simulink model "ignitionScheduler"  (R2020b)
settings: Solver=VariableStepAuto  StartTime=0.0  StopTime=30  RelTol=1e-3
undefined symbols (not defined in the file): I, initialize, T, terminate
libraries: simulink x1, SignalEditorBlockLib x1
settings Model: PauseTimes=75  Creator=Guy  LastModifiedBy=sanumula
settings DataIOCC: SaveOutput=off  DSMLogging=off  SaveTime=off
settings OptimizationCC: UseDivisionForNetSlopeComputation=on
settings DebuggingCC: PregeneratedLibrarySubsystemCodeDiagnostic=none  ArithmeticOperatorsInVariantConditions=warning
settings ModelReferenceCC: EnableRefExpFcnMdlSchedulingChecks=off
settings SFSimCC: SimUseLocalCustomCode=off  CustomCodeUndefinedFunction=UseInterfaceOnly
settings RTWCC: RTWUseLocalCustomCode=off
settings SimscapeCC: SimscapeNormalizeSystem=off  SimscapeLogSimulationStatistics=on  SimscapeLogLimitData=off

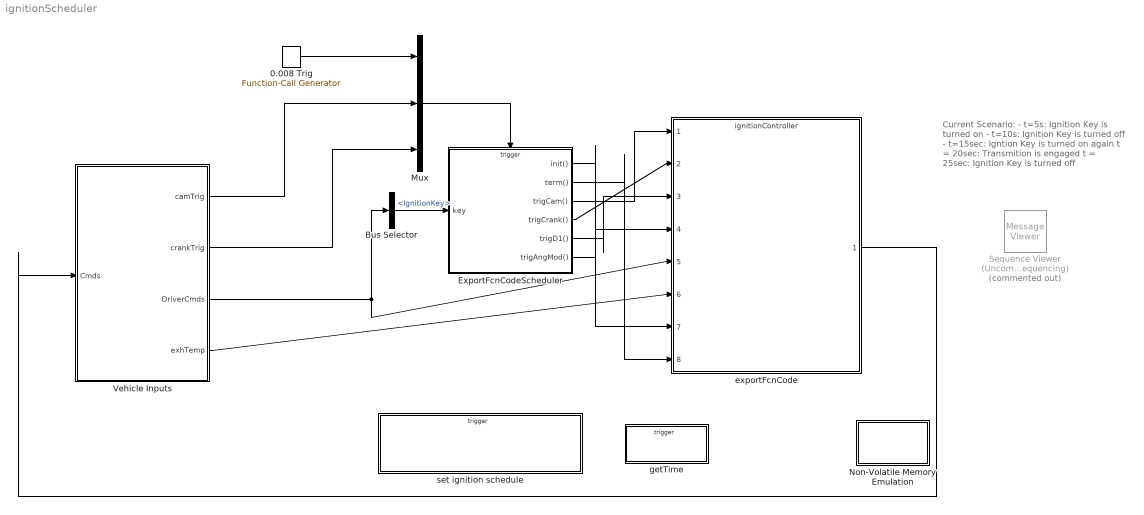
== system ignitionScheduler ==
  note: Current Scenario:
      | - t=5s: Ignition Key is turned on
      | - t=10s: Ignition Key is turned off
      | - t=15sec: Igntion Key is turned on again
      | t = 20sec: Transmition is engaged
      | t = 25sec: Ignition Key is turned off
  0.008 Trig : simulink/Ports & Subsystems/Function-Call Generator  sample_time=.008  numberOfIterations=1  DisallowWideOutput=off
  Bus Selector : BusSelector  OutputSignals=IgnitionKey
  ExportFcnCodeScheduler : Stateflow chart  TreatAsAtomicUnit=on
  Mux : Mux  Inputs=3
  Non-Volatile Memory Emulation : Subsystem
  Sequence Viewer (Uncomment to view events sequencing) : MessageViewer  Commented=on
  Vehicle Inputs : Subsystem
  exportFcnCode : ModelReference  ModelNameDialog=ignitionController.slx  SimulationMode=Normal  ShowModelInitializePort=on  ShowModelTerminatePort=on  ScheduleRates=on  ModelEventPortInfo=I:initialize,T:terminate  ModelReferenceVersion=1.1
  getTime : Subsystem  TreatAsAtomicUnit=on
  set ignition schedule : Subsystem  TreatAsAtomicUnit=on
  wires:
  0.008 Trig/1 -> Mux/1
  Mux/1 -> ExportFcnCodeScheduler/Trigger
  Vehicle Inputs/1(camTrig) -> Mux/2
  Vehicle Inputs/2(crankTrig) -> Mux/3
  Bus Selector/1 -> ExportFcnCodeScheduler/1(key)  "<IgnitionKey>"
  exportFcnCode/1 -> Vehicle Inputs/1(Cmds)
  ExportFcnCodeScheduler/1(init()) -> exportFcnCode/7
  ExportFcnCodeScheduler/2(term()) -> exportFcnCode/8
  ExportFcnCodeScheduler/3(trigCam()) -> exportFcnCode/1
  ExportFcnCodeScheduler/4(trigCrank()) -> exportFcnCode/2
  ExportFcnCodeScheduler/5(trigD1()) -> exportFcnCode/3
  Vehicle Inputs/3(DriverCmds) -> Bus Selector/1, exportFcnCode/5
  Vehicle Inputs/4(exhTemp) -> exportFcnCode/6
  ExportFcnCodeScheduler/6(trigAngMod()) -> exportFcnCode/4

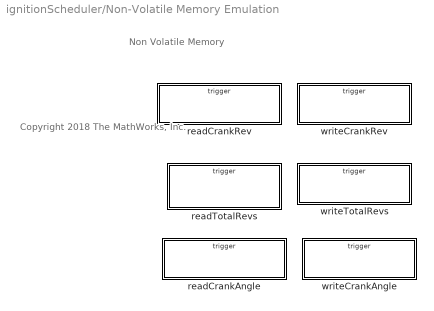
== system ignitionScheduler/Non-Volatile Memory Emulation ==
  note: Copyright 2018 The MathWorks, Inc.
  note: Non Volatile Memory
  readCrankAngle : Subsystem  TreatAsAtomicUnit=on
  readCrankRev : Subsystem  TreatAsAtomicUnit=on
  readTotalRevs : Subsystem  TreatAsAtomicUnit=on
  writeCrankAngle : Subsystem  TreatAsAtomicUnit=on
  writeCrankRev : Subsystem  TreatAsAtomicUnit=on
  writeTotalRevs : Subsystem  TreatAsAtomicUnit=on

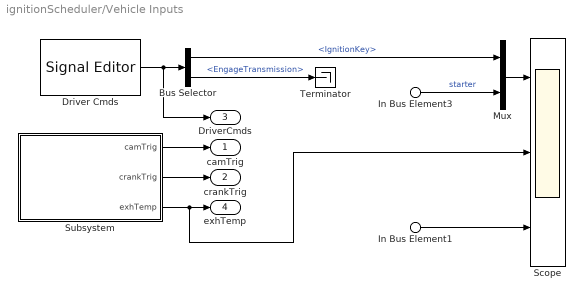
== system ignitionScheduler/Vehicle Inputs ==
  In Bus Element1 : Inport  PortName=Cmds  Element=throttle
  In Bus Element3 : Inport  PortName=Cmds  Element=starter
  Bus Selector : BusSelector  OutputSignals=IgnitionKey,EngageTransmission
  Driver Cmds : SignalEditorBlockLib/Signal Editor  FileName=inputScenarios.mat  ActiveScenario=StartStopTwice  ActiveSignal=CmdBus  IsBus=on  OutputBusObjectStr=Bus: opCmdBus  SampleTime=0  Interpolate=off  ZeroCross=off  OutputAfterFinalValue=Setting to zero  Unit=inherit  PreserveSignalName=on
  Mux : Mux  Inputs=2
  Scope : Scope  NumInputPorts=3
  Subsystem : Subsystem
  Terminator : Terminator
  camTrig : Outport  VectorParamsAs1DForOutWhenUnconnected=off
  crankTrig : Outport  Port=2  VectorParamsAs1DForOutWhenUnconnected=off
  DriverCmds : Outport  Port=3  VectorParamsAs1DForOutWhenUnconnected=off
  exhTemp : Outport  Port=4  VectorParamsAs1DForOutWhenUnconnected=off
  wires:
  Driver Cmds/1 -> DriverCmds/1, Bus Selector/1
  Bus Selector/2 -> Terminator/1  "<EngageTransmission>"
  Mux/1 -> Scope/1
  In Bus Element1/1 -> Scope/3
  In Bus Element3/1 -> Mux/2  "starter"
  Bus Selector/1 -> Mux/1  "<IgnitionKey>"
  Subsystem/1(camTrig) -> camTrig/1
  Subsystem/2(crankTrig) -> crankTrig/1
  Subsystem/3(exhTemp) -> Scope/2, exhTemp/1

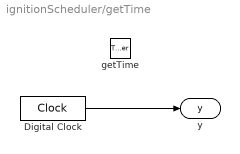
== system ignitionScheduler/getTime ==
  getTime : TriggerPort  TriggerType=function-call  IsSimulinkFunction=on  FunctionName=getTime  VariantControl=(inherit)
  Digital Clock : DigitalClock  SampleTime=-1
  y : ArgOut  DisableCoverage=on  ArgumentName=y
  wires:
  Digital Clock/1 -> y/1

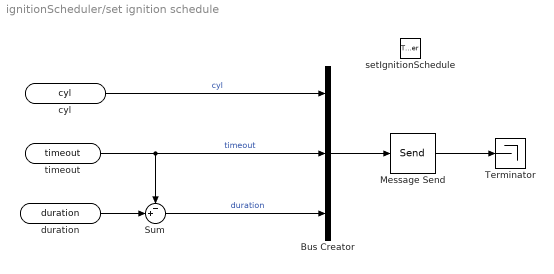
== system ignitionScheduler/set ignition schedule ==
  setIgnitionSchedule : TriggerPort  TriggerType=function-call  IsSimulinkFunction=on  FunctionName=setIgnitionSchedule  VariantControl=(inherit)
  Bus Creator : BusCreator  Inputs=3  OutDataTypeStr=Bus: timerBus  NonVirtualBus=on
  Message Send : Send  OutputPortMessageModes=m
  Sum : Sum  Inputs=-+|
  Terminator : Terminator
  cyl : ArgIn  ArgumentName=cyl
  timeout : ArgIn  DisableCoverage=on  Port=2  ArgumentName=timeout
  duration : ArgIn  Port=3  ArgumentName=duration
  wires:
  Message Send/1 -> Terminator/1
  cyl/1 -> Bus Creator/1  "cyl"
  Sum/1 -> Bus Creator/3  "duration"
  duration/1 -> Sum/2
  timeout/1 -> Sum/1, Bus Creator/2  "timeout"
  Bus Creator/1 -> Message Send/1

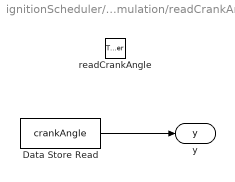
== system ignitionScheduler/Non-Volatile Memory Emulation/readCrankAngle ==
  readCrankAngle : TriggerPort  TriggerType=function-call  IsSimulinkFunction=on  FunctionName=readCrankAngle  VariantControl=(inherit)
  Data Store Read : DataStoreRead  DataStoreName=crankAngle
  y : ArgOut  DisableCoverage=on  ArgumentName=y
  wires:
  Data Store Read/1 -> y/1

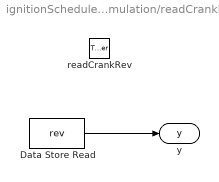
== system ignitionScheduler/Non-Volatile Memory Emulation/readCrankRev ==
  readCrankRev : TriggerPort  TriggerType=function-call  IsSimulinkFunction=on  FunctionName=readCrankRev  VariantControl=(inherit)
  Data Store Read : DataStoreRead  DataStoreName=rev
  y : ArgOut  DisableCoverage=on  OutDataTypeStr=boolean  ArgumentName=y
  wires:
  Data Store Read/1 -> y/1

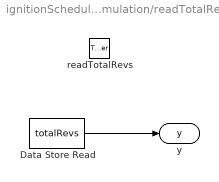
== system ignitionScheduler/Non-Volatile Memory Emulation/readTotalRevs ==
  readTotalRevs : TriggerPort  TriggerType=function-call  IsSimulinkFunction=on  FunctionName=readTotalRevs  VariantControl=(inherit)
  Data Store Read : DataStoreRead  DataStoreName=totalRevs
  y : ArgOut  DisableCoverage=on  ArgumentName=y
  wires:
  Data Store Read/1 -> y/1

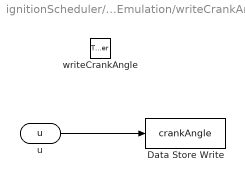
== system ignitionScheduler/Non-Volatile Memory Emulation/writeCrankAngle ==
  writeCrankAngle : TriggerPort  TriggerType=function-call  IsSimulinkFunction=on  FunctionName=writeCrankAngle  VariantControl=(inherit)
  Data Store Write : DataStoreWrite  DataStoreName=crankAngle
  u : ArgIn  DisableCoverage=on  ArgumentName=u
  wires:
  u/1 -> Data Store Write/1

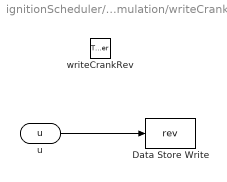
== system ignitionScheduler/Non-Volatile Memory Emulation/writeCrankRev ==
  writeCrankRev : TriggerPort  TriggerType=function-call  IsSimulinkFunction=on  FunctionName=writeCrankRev  VariantControl=(inherit)
  Data Store Write : DataStoreWrite  DataStoreName=rev
  u : ArgIn  DisableCoverage=on  OutDataTypeStr=boolean  ArgumentName=u
  wires:
  u/1 -> Data Store Write/1

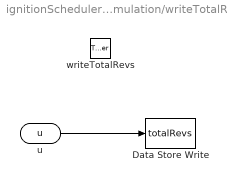
== system ignitionScheduler/Non-Volatile Memory Emulation/writeTotalRevs ==
  writeTotalRevs : TriggerPort  TriggerType=function-call  IsSimulinkFunction=on  FunctionName=writeTotalRevs  VariantControl=(inherit)
  Data Store Write : DataStoreWrite  DataStoreName=totalRevs
  u : ArgIn  DisableCoverage=on  ArgumentName=u
  wires:
  u/1 -> Data Store Write/1

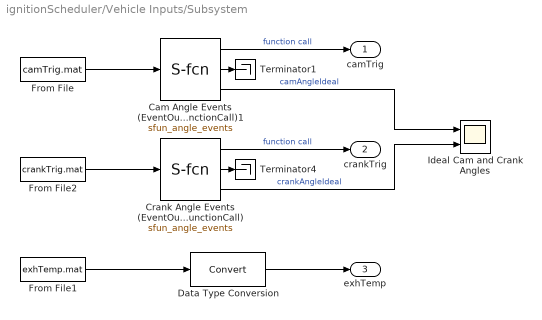
== system ignitionScheduler/Vehicle Inputs/Subsystem ==
  Cam Angle Events (EventOutputType: FunctionCall)1 : S-Function  LoadFcn=|  FunctionName=sfun_angle_events  Parameters=CrossingAngles, InitialAngle, eventOutputType, clockwiseOnly  SFunctionDeploymentMode=off  EnableBusSupport=off  mask(AnglularIntegratorWithEventDetection){CrossingAngles=[0 ], InitialAngle=320, EventOutputType=Function Call, ClockwiseOnly=on}
      | DVG.Registry.registerIcon(...
      | 'BlockIcon.SFunAngleEvents', ...
      | fullfile(matlabroot,'toolbox','simulink','simdemos','simfeatures','slexToothedWheel.svg'))
      mask prompts: CrossingAngles "Crossing Angles:"; InitialAngle "Initial Angle:"; EventOutputType "Event output type:"; ClockwiseOnly "Assume clockwise rotation only"
      mask help:
      | This block integrates the angular velocity input to compute the angle and to fire events at the specified crossing angles. All angles are in degrees, with 0 at the top, incresing clockwise.
      |
      | The crossings angles should be specified as a monotonically increasing vector, with the first element set to 0 and the last element being less than 360 degrees.
      |
      | The first output is a function call, which is fired when an angle crossing event is detected.
      |
      | The second output indicates the direction of the angle crossing event, true for clockwise and false for anti-clockwise.
      |
      | The third output is the angle, wrapped to be in [0, 360) degrees.
      mask init:
      | clockwiseOnly = isequal(get_param(gcb,'ClockwiseOnly'),'on');
      | 
      | switch get_param(gcb,'EventOutputType')
      |     case 'Trigger Pulse'
      |         eventOutputType = 0;
      |     case 'Function Call'
      |         eventOutputType = 1;
      |     otherwise
      |         eventOutputType = 2;
      | end
      mask TypeOptions EventOutputType: Trigger Pulse | Function Call
      mask Display: %image('slexToothedWheel.svg');
  Crank Angle Events (EventOutputType: FunctionCall) : S-Function  LoadFcn=|  FunctionName=sfun_angle_events  Parameters=CrossingAngles, InitialAngle, eventOutputType, clockwiseOnly  SFunctionDeploymentMode=off  EnableBusSupport=off  mask(AnglularIntegratorWithEventDetection){CrossingAngles=[0:10:340], InitialAngle=0, EventOutputType=Function Call, ClockwiseOnly=on}
      | DVG.Registry.registerIcon(...
      | 'BlockIcon.SFunAngleEvents', ...
      | fullfile(matlabroot,'toolbox','simulink','simdemos','simfeatures','slexToothedWheel.svg'))
      mask prompts: CrossingAngles "Crossing Angles:"; InitialAngle "Initial Angle:"; EventOutputType "Event output type:"; ClockwiseOnly "Assume clockwise rotation only"
      mask help:
      | This block integrates the angular velocity input to compute the angle and to fire events at the specified crossing angles. All angles are in degrees, with 0 at the top, incresing clockwise.
      |
      | The crossings angles should be specified as a monotonically increasing vector, with the first element set to 0 and the last element being less than 360 degrees.
      |
      | The first output is a function call, which is fired when an angle crossing event is detected.
      |
      | The second output indicates the direction of the angle crossing event, true for clockwise and false for anti-clockwise.
      |
      | The third output is the angle, wrapped to be in [0, 360) degrees.
      mask init: same as ignitionScheduler/Vehicle Inputs/Subsystem/Cam Angle Events (EventOutputType: FunctionCall)1
      mask TypeOptions EventOutputType: Trigger Pulse | Function Call
      mask Display: %image('slexToothedWheel.svg');
  Data Type Conversion : DataTypeConversion
  From File : FromFile  FileName=camTrig.mat  SampleTime=0
  From File1 : FromFile  FileName=exhTemp.mat  SampleTime=0
  From File2 : FromFile  FileName=crankTrig.mat  SampleTime=0
  Ideal Cam and Crank Angles : Scope  NumInputPorts=2
  Terminator1 : Terminator
  Terminator4 : Terminator
  camTrig : Outport  VectorParamsAs1DForOutWhenUnconnected=off
  crankTrig : Outport  Port=2  VectorParamsAs1DForOutWhenUnconnected=off
  exhTemp : Outport  Port=3
  wires:
  Crank Angle Events (EventOutputType: FunctionCall)/2 -> Terminator4/1
  Crank Angle Events (EventOutputType: FunctionCall)/1 -> crankTrig/1  "function call"
  Cam Angle Events (EventOutputType: FunctionCall)1/1 -> camTrig/1  "function call"
  Crank Angle Events (EventOutputType: FunctionCall)/3 -> Ideal Cam and Crank Angles/2  "crankAngleIdeal"
  From File2/1 -> Crank Angle Events (EventOutputType: FunctionCall)/1
  Cam Angle Events (EventOutputType: FunctionCall)1/2 -> Terminator1/1
  Cam Angle Events (EventOutputType: FunctionCall)1/3 -> Ideal Cam and Crank Angles/1  "camAngleIdeal"
  From File/1 -> Cam Angle Events (EventOutputType: FunctionCall)1/1
  From File1/1 -> Data Type Conversion/1
  Data Type Conversion/1 -> exhTemp/1

== stateflow chart ignitionScheduler/ExportFcnCodeScheduler ==
  state Off
  note: Assumption:
      | As simplification, I assume that as soon as the key is turned on, the ECU is powered on.
      | For shutdown, the ECU will read the key and do some work before shutting down and updating "isECUPowered".
  state Running
    entry: isECUPowered = true; init();
    on every(1, cam): trigCam();
    on every(1, crank): trigCrank();
    on every(1, crank): trigAngMod();
    on every(1, D1): trigD1();
    exit: term();
  (default) -> Off : {isECUPowered = false;}
  Off -> Running : [key == true]
  Running -> Off : [isECUPowered == false]
  data: key input boolean size=1; isECUPowered data_store_memory
  events: D1 input FUNCTION_CALL_EVENT; cam input FUNCTION_CALL_EVENT; crank input FUNCTION_CALL_EVENT; init output FUNCTION_CALL_EVENT; term output FUNCTION_CALL_EVENT; trigCam output FUNCTION_CALL_EVENT; trigCrank output FUNCTION_CALL_EVENT; trigD1 output FUNCTION_CALL_EVENT; trigAngMod output FUNCTION_CALL_EVENT
